simulink library "calc_Lap_Average"  (R2020a)
settings: Solver=VariableStepAuto  StartTime=0.0  StopTime=10.0  RelTol=1e-3
libraries: dspsigops x2
settings Model: Creator=Ayaz  LastModifiedBy=Ayaz

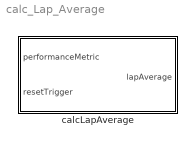
== system calc_Lap_Average ==
  calcLapAverage : Subsystem

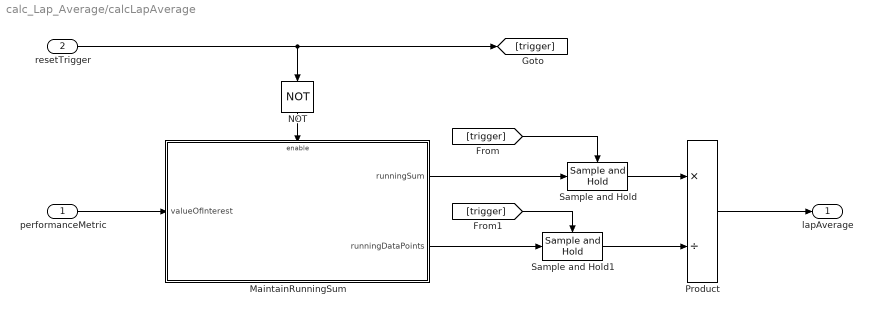
== system calc_Lap_Average/calcLapAverage ==
  performanceMetric : Inport
  resetTrigger : Inport  Port=2
  MaintainRunningSum : Subsystem  TreatAsAtomicUnit=on
  NOT : Logic  Operator=NOT  IconShape=distinctive  AllPortsSameDT=off  OutDataTypeStr=boolean
  Product : Product  Inputs=*/
  Sample and Hold : dspsigops/Sample and Hold  trig=Rising edge  initCond=0  latchinput=off
  Sample and Hold1 : dspsigops/Sample and Hold  trig=Rising edge  initCond=1  latchinput=off
  lapAverage : Outport
  wires:
  performanceMetric/1 -> MaintainRunningSum/1(valueOfInterest)
  MaintainRunningSum/1(runningSum) -> Sample and Hold/1
  MaintainRunningSum/2(runningDataPoints) -> Sample and Hold1/1
  [trigger] -> Sample and Hold/Trigger
  [trigger] -> Sample and Hold1/Trigger
  Sample and Hold/1 -> Product/1
  Sample and Hold1/1 -> Product/2
  Product/1 -> lapAverage/1
  resetTrigger/1 -> NOT/1, [trigger]
  NOT/1 -> MaintainRunningSum/Enable

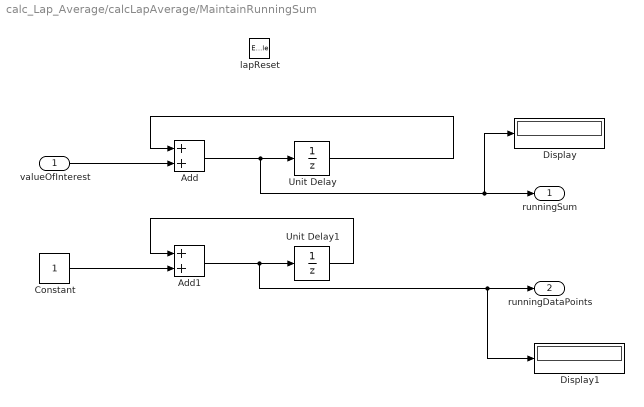
== system calc_Lap_Average/calcLapAverage/MaintainRunningSum ==
  valueOfInterest : Inport
  lapReset : EnablePort  StatesWhenEnabling=reset
  Add : Sum
  Add1 : Sum
  Constant : Constant
  Display : Display
  Display1 : Display
  Unit Delay : UnitDelay  SampleTime=-1  HasFrameUpgradeWarning=on
  Unit Delay1 : UnitDelay  SampleTime=-1  HasFrameUpgradeWarning=on
  runningSum : Outport
  runningDataPoints : Outport  Port=2
  wires:
  Add/1 -> Unit Delay/1, Display/1, runningSum/1
  Unit Delay/1 -> Add/1
  valueOfInterest/1 -> Add/2
  Constant/1 -> Add1/2
  Add1/1 -> Display1/1, runningDataPoints/1, Unit Delay1/1
  Unit Delay1/1 -> Add1/1
